simulink model "SecRwRtStLgrstInwdOtwdTrgtPosSelc"  (R2018b)
settings: Solver=FixedStepDiscrete  StartTime=0.0  StopTime=10.0  FixedStep=0.01  RelTol=1e-3
undefined symbols (not defined in the file or in its folder): KeSMSw4SAcsMd24SecRwRtStLegrstOtwdInwdPos_Val, KeSMSw4SAcsMd24SecRwRtStLegrstOtwdInwdPosMax_Val, KeSMSw4SAcsMd24SecRwRtStLegrstOtwdInwdPosMin_Val, KeSMSw4SAcsMd26SecRwRtStLegrstOtwdInwdPos_Val, KeSMSw4SAcsMd26SecRwRtStLegrstOtwdInwdPosMax_Val, KeSMSw4SAcsMd26SecRwRtStLegrstOtwdInwdPosMin_Val, KeSMSw4SLegrstCloseMdSecRwRtStLgrstOtwdInwdPos_Val, KeSMSw4SLegrstCloseMdSecRwRtStLgrstOtwdInwdPosMax_Val, KeSMSw4SLegrstCloseMdSecRwRtStLgrstOtwdInwdPosMin_Val, KeSMSw4SLegrstOpenMdSecRwRtStLgrstOtwdInwdPos_Val, KeSMSw4SLegrstOpenMdSecRwRtStLgrstOtwdInwdPosMax_Val, KeSMSw4SLegrstOpenMdSecRwRtStLgrstOtwdInwdPosMin_Val, KeSMSw4sLyingMDSecRwRtStLgrstOtwdInwdPos_160_Val, KeSMSw4sLyingMDSecRwRtStLgrstOtwdInwdPos_165_Val, KeSMSw4sLyingMDSecRwRtStLgrstOtwdInwdPos_170_Val, KeSMSw4sLyingMDSecRwRtStLgrstOtwdInwdPos_175_Val, KeSMSw4sLyingMDSecRwRtStLgrstOtwdInwdPos_180_Val, KeSMSw4sLyingMDSecRwRtStLgrstOtwdInwdPos_Below160_Val, KeSMSw4sLyingMDSecRwRtStLgrstOtwdInwdPos_Over180_Val, KeSMSw4sLyingMDSecRwRtStLgrstOtwdInwdPosMax_160_Val, KeSMSw4sLyingMDSecRwRtStLgrstOtwdInwdPosMax_165_Val, KeSMSw4sLyingMDSecRwRtStLgrstOtwdInwdPosMax_170_Val, KeSMSw4sLyingMDSecRwRtStLgrstOtwdInwdPosMax_175_Val, KeSMSw4sLyingMDSecRwRtStLgrstOtwdInwdPosMax_180_Val, KeSMSw4sLyingMDSecRwRtStLgrstOtwdInwdPosMax_Below160_Val, KeSMSw4sLyingMDSecRwRtStLgrstOtwdInwdPosMax_Over180_Val, KeSMSw4sLyingMDSecRwRtStLgrstOtwdInwdPosMin_160_Val, KeSMSw4sLyingMDSecRwRtStLgrstOtwdInwdPosMin_165_Val, KeSMSw4sLyingMDSecRwRtStLgrstOtwdInwdPosMin_170_Val, KeSMSw4sLyingMDSecRwRtStLgrstOtwdInwdPosMin_175_Val, KeSMSw4sLyingMDSecRwRtStLgrstOtwdInwdPosMin_180_Val, KeSMSw4sLyingMDSecRwRtStLgrstOtwdInwdPosMin_Below160_Val, KeSMSw4sLyingMDSecRwRtStLgrstOtwdInwdPosMin_Over180_Val, KeSMSw4sRecoveryMDSecRwRtStLgrstOtwdInwdPos_160_Val, KeSMSw4sRecoveryMDSecRwRtStLgrstOtwdInwdPos_165_Val, KeSMSw4sRecoveryMDSecRwRtStLgrstOtwdInwdPos_170_Val, KeSMSw4sRecoveryMDSecRwRtStLgrstOtwdInwdPos_175_Val, KeSMSw4sRecoveryMDSecRwRtStLgrstOtwdInwdPos_180_Val, KeSMSw4sRecoveryMDSecRwRtStLgrstOtwdInwdPos_Below160_Val, KeSMSw4sRecoveryMDSecRwRtStLgrstOtwdInwdPos_Over180_Val, KeSMSw4sRecoveryMDSecRwRtStLgrstOtwdInwdPosMax_160_Val, KeSMSw4sRecoveryMDSecRwRtStLgrstOtwdInwdPosMax_165_Val, KeSMSw4sRecoveryMDSecRwRtStLgrstOtwdInwdPosMax_170_Val, KeSMSw4sRecoveryMDSecRwRtStLgrstOtwdInwdPosMax_175_Val, KeSMSw4sRecoveryMDSecRwRtStLgrstOtwdInwdPosMax_180_Val, KeSMSw4sRecoveryMDSecRwRtStLgrstOtwdInwdPosMax_Below160_Val, KeSMSw4sRecoveryMDSecRwRtStLgrstOtwdInwdPosMax_Over180_Val, KeSMSw4sRecoveryMDSecRwRtStLgrstOtwdInwdPosMin_160_Val, KeSMSw4sRecoveryMDSecRwRtStLgrstOtwdInwdPosMin_165_Val, KeSMSw4sRecoveryMDSecRwRtStLgrstOtwdInwdPosMin_170_Val, KeSMSw4sRecoveryMDSecRwRtStLgrstOtwdInwdPosMin_175_Val, KeSMSw4sRecoveryMDSecRwRtStLgrstOtwdInwdPosMin_180_Val, KeSMSw4sRecoveryMDSecRwRtStLgrstOtwdInwdPosMin_Below160_Val, KeSMSw4sRecoveryMDSecRwRtStLgrstOtwdInwdPosMin_Over180_Val, KeSMSw4sVIPMDSecRwRtStLgrstOtwdInwdPos_160_Val, KeSMSw4sVIPMDSecRwRtStLgrstOtwdInwdPos_165_Val, KeSMSw4sVIPMDSecRwRtStLgrstOtwdInwdPos_170_Val, KeSMSw4sVIPMDSecRwRtStLgrstOtwdInwdPos_175_Val, KeSMSw4sVIPMDSecRwRtStLgrstOtwdInwdPos_180_Val, KeSMSw4sVIPMDSecRwRtStLgrstOtwdInwdPos_Below160_Val ... (+40)
libraries: TrgtPosSelcLib x10
(part 2 of 2)

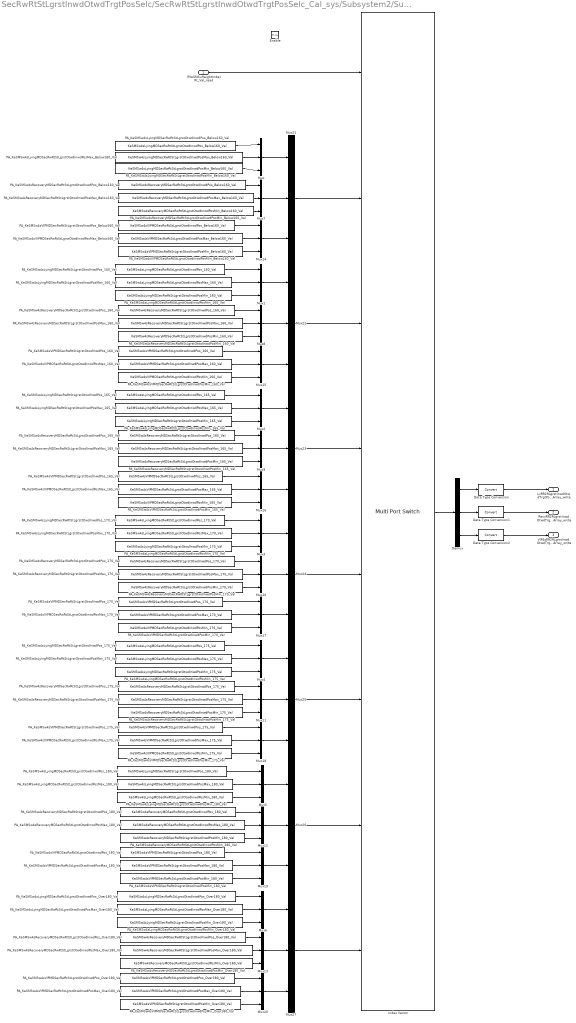
== system SecRwRtStLgrstInwdOtwdTrgtPosSelc/SecRwRtStLgrstInwdOtwdTrgtPosSelc_Cal_sys/Subsystem2/Subsystem ==
  IfVeSMSuHeightIndexRt_Val_read : Inport
  Enable : EnablePort
  Data Type Conversion : DataTypeConversion
  Data Type Conversion1 : DataTypeConversion
  Data Type Conversion2 : DataTypeConversion
  Demux : Demux  Outputs=3
  Index Vector : MultiPortSwitch  DataPortOrder=Zero-based contiguous  Inputs=7  zeroidx=on
  Mux{,1..27} (28 alike) : Mux  Inputs=3
  PA_KeSMSw4sLyingMDSecRwRtStLgrstOtwdInwdPosMax_160_Val : Constant  Value=KeSMSw4sLyingMDSecRwRtStLgrstOtwdInwdPosMax_160_Val
  PA_KeSMSw4sLyingMDSecRwRtStLgrstOtwdInwdPosMax_165_Val : Constant  Value=KeSMSw4sLyingMDSecRwRtStLgrstOtwdInwdPosMax_165_Val
  PA_KeSMSw4sLyingMDSecRwRtStLgrstOtwdInwdPosMax_170_Val : Constant  Value=KeSMSw4sLyingMDSecRwRtStLgrstOtwdInwdPosMax_170_Val
  PA_KeSMSw4sLyingMDSecRwRtStLgrstOtwdInwdPosMax_175_Val : Constant  Value=KeSMSw4sLyingMDSecRwRtStLgrstOtwdInwdPosMax_175_Val
  PA_KeSMSw4sLyingMDSecRwRtStLgrstOtwdInwdPosMax_180_Val : Constant  Value=KeSMSw4sLyingMDSecRwRtStLgrstOtwdInwdPosMax_180_Val
  PA_KeSMSw4sLyingMDSecRwRtStLgrstOtwdInwdPosMax_Below160_Val : Constant  Value=KeSMSw4sLyingMDSecRwRtStLgrstOtwdInwdPosMax_Below160_Val
  PA_KeSMSw4sLyingMDSecRwRtStLgrstOtwdInwdPosMax_Over180_Val : Constant  Value=KeSMSw4sLyingMDSecRwRtStLgrstOtwdInwdPosMax_Over180_Val
  PA_KeSMSw4sLyingMDSecRwRtStLgrstOtwdInwdPosMin_160_Val : Constant  Value=KeSMSw4sLyingMDSecRwRtStLgrstOtwdInwdPosMin_160_Val
  PA_KeSMSw4sLyingMDSecRwRtStLgrstOtwdInwdPosMin_165_Val : Constant  Value=KeSMSw4sLyingMDSecRwRtStLgrstOtwdInwdPosMin_165_Val
  PA_KeSMSw4sLyingMDSecRwRtStLgrstOtwdInwdPosMin_170_Val : Constant  Value=KeSMSw4sLyingMDSecRwRtStLgrstOtwdInwdPosMin_170_Val
  PA_KeSMSw4sLyingMDSecRwRtStLgrstOtwdInwdPosMin_175_Val : Constant  Value=KeSMSw4sLyingMDSecRwRtStLgrstOtwdInwdPosMin_175_Val
  PA_KeSMSw4sLyingMDSecRwRtStLgrstOtwdInwdPosMin_180_Val : Constant  Value=KeSMSw4sLyingMDSecRwRtStLgrstOtwdInwdPosMin_180_Val
  PA_KeSMSw4sLyingMDSecRwRtStLgrstOtwdInwdPosMin_Below160_Val : Constant  Value=KeSMSw4sLyingMDSecRwRtStLgrstOtwdInwdPosMin_Below160_Val
  PA_KeSMSw4sLyingMDSecRwRtStLgrstOtwdInwdPosMin_Over180_Val : Constant  Value=KeSMSw4sLyingMDSecRwRtStLgrstOtwdInwdPosMin_Over180_Val
  PA_KeSMSw4sLyingMDSecRwRtStLgrstOtwdInwdPos_160_Val : Constant  Value=KeSMSw4sLyingMDSecRwRtStLgrstOtwdInwdPos_160_Val
  PA_KeSMSw4sLyingMDSecRwRtStLgrstOtwdInwdPos_165_Val : Constant  Value=KeSMSw4sLyingMDSecRwRtStLgrstOtwdInwdPos_165_Val
  PA_KeSMSw4sLyingMDSecRwRtStLgrstOtwdInwdPos_170_Val : Constant  Value=KeSMSw4sLyingMDSecRwRtStLgrstOtwdInwdPos_170_Val
  PA_KeSMSw4sLyingMDSecRwRtStLgrstOtwdInwdPos_175_Val : Constant  Value=KeSMSw4sLyingMDSecRwRtStLgrstOtwdInwdPos_175_Val
  PA_KeSMSw4sLyingMDSecRwRtStLgrstOtwdInwdPos_180_Val : Constant  Value=KeSMSw4sLyingMDSecRwRtStLgrstOtwdInwdPos_180_Val
  PA_KeSMSw4sLyingMDSecRwRtStLgrstOtwdInwdPos_Below160_Val : Constant  Value=KeSMSw4sLyingMDSecRwRtStLgrstOtwdInwdPos_Below160_Val
  PA_KeSMSw4sLyingMDSecRwRtStLgrstOtwdInwdPos_Over180_Val : Constant  Value=KeSMSw4sLyingMDSecRwRtStLgrstOtwdInwdPos_Over180_Val
  PA_KeSMSw4sRecoveryMDSecRwRtStLgrstOtwdInwdPosMax_160_Val : Constant  Value=KeSMSw4sRecoveryMDSecRwRtStLgrstOtwdInwdPosMax_160_Val
  PA_KeSMSw4sRecoveryMDSecRwRtStLgrstOtwdInwdPosMax_165_Val : Constant  Value=KeSMSw4sRecoveryMDSecRwRtStLgrstOtwdInwdPosMax_165_Val
  PA_KeSMSw4sRecoveryMDSecRwRtStLgrstOtwdInwdPosMax_170_Val : Constant  Value=KeSMSw4sRecoveryMDSecRwRtStLgrstOtwdInwdPosMax_170_Val
  PA_KeSMSw4sRecoveryMDSecRwRtStLgrstOtwdInwdPosMax_175_Val : Constant  Value=KeSMSw4sRecoveryMDSecRwRtStLgrstOtwdInwdPosMax_175_Val
  PA_KeSMSw4sRecoveryMDSecRwRtStLgrstOtwdInwdPosMax_180_Val : Constant  Value=KeSMSw4sRecoveryMDSecRwRtStLgrstOtwdInwdPosMax_180_Val
  PA_KeSMSw4sRecoveryMDSecRwRtStLgrstOtwdInwdPosMax_Below160_Val : Constant  Value=KeSMSw4sRecoveryMDSecRwRtStLgrstOtwdInwdPosMax_Below160_Val
  PA_KeSMSw4sRecoveryMDSecRwRtStLgrstOtwdInwdPosMax_Over180_Val : Constant  Value=KeSMSw4sRecoveryMDSecRwRtStLgrstOtwdInwdPosMax_Over180_Val
  PA_KeSMSw4sRecoveryMDSecRwRtStLgrstOtwdInwdPosMin_160_Val : Constant  Value=KeSMSw4sRecoveryMDSecRwRtStLgrstOtwdInwdPosMin_160_Val
  PA_KeSMSw4sRecoveryMDSecRwRtStLgrstOtwdInwdPosMin_165_Val : Constant  Value=KeSMSw4sRecoveryMDSecRwRtStLgrstOtwdInwdPosMin_165_Val
  PA_KeSMSw4sRecoveryMDSecRwRtStLgrstOtwdInwdPosMin_170_Val : Constant  Value=KeSMSw4sRecoveryMDSecRwRtStLgrstOtwdInwdPosMin_170_Val
  PA_KeSMSw4sRecoveryMDSecRwRtStLgrstOtwdInwdPosMin_175_Val : Constant  Value=KeSMSw4sRecoveryMDSecRwRtStLgrstOtwdInwdPosMin_175_Val
  PA_KeSMSw4sRecoveryMDSecRwRtStLgrstOtwdInwdPosMin_180_Val : Constant  Value=KeSMSw4sRecoveryMDSecRwRtStLgrstOtwdInwdPosMin_180_Val
  PA_KeSMSw4sRecoveryMDSecRwRtStLgrstOtwdInwdPosMin_Below160_Val : Constant  Value=KeSMSw4sRecoveryMDSecRwRtStLgrstOtwdInwdPosMin_Below160_Val
  PA_KeSMSw4sRecoveryMDSecRwRtStLgrstOtwdInwdPosMin_Over180_Val : Constant  Value=KeSMSw4sRecoveryMDSecRwRtStLgrstOtwdInwdPosMin_Over180_Val
  PA_KeSMSw4sRecoveryMDSecRwRtStLgrstOtwdInwdPos_160_Val : Constant  Value=KeSMSw4sRecoveryMDSecRwRtStLgrstOtwdInwdPos_160_Val
  PA_KeSMSw4sRecoveryMDSecRwRtStLgrstOtwdInwdPos_165_Val : Constant  Value=KeSMSw4sRecoveryMDSecRwRtStLgrstOtwdInwdPos_165_Val
  PA_KeSMSw4sRecoveryMDSecRwRtStLgrstOtwdInwdPos_170_Val : Constant  Value=KeSMSw4sRecoveryMDSecRwRtStLgrstOtwdInwdPos_170_Val
  PA_KeSMSw4sRecoveryMDSecRwRtStLgrstOtwdInwdPos_175_Val : Constant  Value=KeSMSw4sRecoveryMDSecRwRtStLgrstOtwdInwdPos_175_Val
  PA_KeSMSw4sRecoveryMDSecRwRtStLgrstOtwdInwdPos_180_Val : Constant  Value=KeSMSw4sRecoveryMDSecRwRtStLgrstOtwdInwdPos_180_Val
  PA_KeSMSw4sRecoveryMDSecRwRtStLgrstOtwdInwdPos_Below160_Val : Constant  Value=KeSMSw4sRecoveryMDSecRwRtStLgrstOtwdInwdPos_Below160_Val
  PA_KeSMSw4sRecoveryMDSecRwRtStLgrstOtwdInwdPos_Over180_Val : Constant  Value=KeSMSw4sRecoveryMDSecRwRtStLgrstOtwdInwdPos_Over180_Val
  PA_KeSMSw4sVIPMDSecRwRtStLgrstOtwdInwdPosMax_160_Val : Constant  Value=KeSMSw4sVIPMDSecRwRtStLgrstOtwdInwdPosMax_160_Val
  PA_KeSMSw4sVIPMDSecRwRtStLgrstOtwdInwdPosMax_165_Val : Constant  Value=KeSMSw4sVIPMDSecRwRtStLgrstOtwdInwdPosMax_165_Val
  PA_KeSMSw4sVIPMDSecRwRtStLgrstOtwdInwdPosMax_170_Val : Constant  Value=KeSMSw4sVIPMDSecRwRtStLgrstOtwdInwdPosMax_170_Val
  PA_KeSMSw4sVIPMDSecRwRtStLgrstOtwdInwdPosMax_175_Val : Constant  Value=KeSMSw4sVIPMDSecRwRtStLgrstOtwdInwdPosMax_175_Val
  PA_KeSMSw4sVIPMDSecRwRtStLgrstOtwdInwdPosMax_180_Val : Constant  Value=KeSMSw4sVIPMDSecRwRtStLgrstOtwdInwdPosMax_180_Val
  PA_KeSMSw4sVIPMDSecRwRtStLgrstOtwdInwdPosMax_Below160_Val : Constant  Value=KeSMSw4sVIPMDSecRwRtStLgrstOtwdInwdPosMax_Below160_Val
  PA_KeSMSw4sVIPMDSecRwRtStLgrstOtwdInwdPosMax_Over180_Val : Constant  Value=KeSMSw4sVIPMDSecRwRtStLgrstOtwdInwdPosMax_Over180_Val
  PA_KeSMSw4sVIPMDSecRwRtStLgrstOtwdInwdPosMin_160_Val : Constant  Value=KeSMSw4sVIPMDSecRwRtStLgrstOtwdInwdPosMin_160_Val
  PA_KeSMSw4sVIPMDSecRwRtStLgrstOtwdInwdPosMin_165_Val : Constant  Value=KeSMSw4sVIPMDSecRwRtStLgrstOtwdInwdPosMin_165_Val
  PA_KeSMSw4sVIPMDSecRwRtStLgrstOtwdInwdPosMin_170_Val : Constant  Value=KeSMSw4sVIPMDSecRwRtStLgrstOtwdInwdPosMin_170_Val
  PA_KeSMSw4sVIPMDSecRwRtStLgrstOtwdInwdPosMin_175_Val : Constant  Value=KeSMSw4sVIPMDSecRwRtStLgrstOtwdInwdPosMin_175_Val
  PA_KeSMSw4sVIPMDSecRwRtStLgrstOtwdInwdPosMin_180_Val : Constant  Value=KeSMSw4sVIPMDSecRwRtStLgrstOtwdInwdPosMin_180_Val
  PA_KeSMSw4sVIPMDSecRwRtStLgrstOtwdInwdPosMin_Below160_Val : Constant  Value=KeSMSw4sVIPMDSecRwRtStLgrstOtwdInwdPosMin_Below160_Val
  PA_KeSMSw4sVIPMDSecRwRtStLgrstOtwdInwdPosMin_Over180_Val : Constant  Value=KeSMSw4sVIPMDSecRwRtStLgrstOtwdInwdPosMin_Over180_Val
  PA_KeSMSw4sVIPMDSecRwRtStLgrstOtwdInwdPos_160_Val : Constant  Value=KeSMSw4sVIPMDSecRwRtStLgrstOtwdInwdPos_160_Val
  PA_KeSMSw4sVIPMDSecRwRtStLgrstOtwdInwdPos_165_Val : Constant  Value=KeSMSw4sVIPMDSecRwRtStLgrstOtwdInwdPos_165_Val
  PA_KeSMSw4sVIPMDSecRwRtStLgrstOtwdInwdPos_170_Val : Constant  Value=KeSMSw4sVIPMDSecRwRtStLgrstOtwdInwdPos_170_Val
  PA_KeSMSw4sVIPMDSecRwRtStLgrstOtwdInwdPos_175_Val : Constant  Value=KeSMSw4sVIPMDSecRwRtStLgrstOtwdInwdPos_175_Val
  PA_KeSMSw4sVIPMDSecRwRtStLgrstOtwdInwdPos_180_Val : Constant  Value=KeSMSw4sVIPMDSecRwRtStLgrstOtwdInwdPos_180_Val
  PA_KeSMSw4sVIPMDSecRwRtStLgrstOtwdInwdPos_Below160_Val : Constant  Value=KeSMSw4sVIPMDSecRwRtStLgrstOtwdInwdPos_Below160_Val
  PA_KeSMSw4sVIPMDSecRwRtStLgrstOtwdInwdPos_Over180_Val : Constant  Value=KeSMSw4sVIPMDSecRwRtStLgrstOtwdInwdPos_Over180_Val
  LyRR2RLgrstInwdOtwdTrgtPosCalib_TrgtPosArray_write : Outport
  RecvRR2RLgrstInwdOtwdTrgtPosCalib_TrgtPosArray_write : Outport  Port=2
  VIP4sRR2RLgrstInwdOtwdTrgtPosCalib_TrgtPosArray_write : Outport  Port=3
  wires:
  Demux/1 -> Data Type Conversion/1
  Demux/2 -> Data Type Conversion1/1
  Demux/3 -> Data Type Conversion2/1
  Data Type Conversion/1 -> LyRR2RLgrstInwdOtwdTrgtPosCalib_TrgtPosArray_write/1
  Data Type Conversion1/1 -> RecvRR2RLgrstInwdOtwdTrgtPosCalib_TrgtPosArray_write/1
  Data Type Conversion2/1 -> VIP4sRR2RLgrstInwdOtwdTrgtPosCalib_TrgtPosArray_write/1
  PA_KeSMSw4sLyingMDSecRwRtStLgrstOtwdInwdPosMax_Below160_Val/1 -> Mux/2
  PA_KeSMSw4sLyingMDSecRwRtStLgrstOtwdInwdPosMin_Below160_Val/1 -> Mux/3
  PA_KeSMSw4sLyingMDSecRwRtStLgrstOtwdInwdPos_Below160_Val/1 -> Mux/1
  PA_KeSMSw4sLyingMDSecRwRtStLgrstOtwdInwdPosMax_160_Val/1 -> Mux1/2
  PA_KeSMSw4sLyingMDSecRwRtStLgrstOtwdInwdPosMin_160_Val/1 -> Mux1/3
  PA_KeSMSw4sLyingMDSecRwRtStLgrstOtwdInwdPos_160_Val/1 -> Mux1/1
  PA_KeSMSw4sLyingMDSecRwRtStLgrstOtwdInwdPosMax_165_Val/1 -> Mux2/2
  PA_KeSMSw4sLyingMDSecRwRtStLgrstOtwdInwdPosMin_165_Val/1 -> Mux2/3
  PA_KeSMSw4sLyingMDSecRwRtStLgrstOtwdInwdPos_165_Val/1 -> Mux2/1
  PA_KeSMSw4sLyingMDSecRwRtStLgrstOtwdInwdPosMax_170_Val/1 -> Mux3/2
  PA_KeSMSw4sLyingMDSecRwRtStLgrstOtwdInwdPosMin_170_Val/1 -> Mux3/3
  PA_KeSMSw4sLyingMDSecRwRtStLgrstOtwdInwdPos_170_Val/1 -> Mux3/1
  PA_KeSMSw4sLyingMDSecRwRtStLgrstOtwdInwdPosMax_175_Val/1 -> Mux4/2
  PA_KeSMSw4sLyingMDSecRwRtStLgrstOtwdInwdPosMin_175_Val/1 -> Mux4/3
  PA_KeSMSw4sLyingMDSecRwRtStLgrstOtwdInwdPos_175_Val/1 -> Mux4/1
  PA_KeSMSw4sLyingMDSecRwRtStLgrstOtwdInwdPosMax_180_Val/1 -> Mux5/2
  PA_KeSMSw4sLyingMDSecRwRtStLgrstOtwdInwdPosMin_180_Val/1 -> Mux5/3
  PA_KeSMSw4sLyingMDSecRwRtStLgrstOtwdInwdPos_180_Val/1 -> Mux5/1
  PA_KeSMSw4sLyingMDSecRwRtStLgrstOtwdInwdPosMax_Over180_Val/1 -> Mux6/2
  PA_KeSMSw4sLyingMDSecRwRtStLgrstOtwdInwdPosMin_Over180_Val/1 -> Mux6/3
  PA_KeSMSw4sLyingMDSecRwRtStLgrstOtwdInwdPos_Over180_Val/1 -> Mux6/1
  IfVeSMSuHeightIndexRt_Val_read/1 -> Index Vector/1
  PA_KeSMSw4sRecoveryMDSecRwRtStLgrstOtwdInwdPos_Below160_Val/1 -> Mux7/1
  PA_KeSMSw4sRecoveryMDSecRwRtStLgrstOtwdInwdPosMax_Below160_Val/1 -> Mux7/2
  PA_KeSMSw4sRecoveryMDSecRwRtStLgrstOtwdInwdPosMin_Below160_Val/1 -> Mux7/3
  PA_KeSMSw4sRecoveryMDSecRwRtStLgrstOtwdInwdPos_160_Val/1 -> Mux8/1
  PA_KeSMSw4sRecoveryMDSecRwRtStLgrstOtwdInwdPosMax_160_Val/1 -> Mux8/2
  PA_KeSMSw4sRecoveryMDSecRwRtStLgrstOtwdInwdPosMin_160_Val/1 -> Mux8/3
  PA_KeSMSw4sRecoveryMDSecRwRtStLgrstOtwdInwdPos_165_Val/1 -> Mux9/1
  PA_KeSMSw4sRecoveryMDSecRwRtStLgrstOtwdInwdPosMax_165_Val/1 -> Mux9/2
  PA_KeSMSw4sRecoveryMDSecRwRtStLgrstOtwdInwdPosMin_165_Val/1 -> Mux9/3
  PA_KeSMSw4sRecoveryMDSecRwRtStLgrstOtwdInwdPos_170_Val/1 -> Mux10/1
  PA_KeSMSw4sRecoveryMDSecRwRtStLgrstOtwdInwdPosMax_170_Val/1 -> Mux10/2
  PA_KeSMSw4sRecoveryMDSecRwRtStLgrstOtwdInwdPosMin_170_Val/1 -> Mux10/3
  PA_KeSMSw4sRecoveryMDSecRwRtStLgrstOtwdInwdPos_175_Val/1 -> Mux11/1
  PA_KeSMSw4sRecoveryMDSecRwRtStLgrstOtwdInwdPosMax_175_Val/1 -> Mux11/2
  PA_KeSMSw4sRecoveryMDSecRwRtStLgrstOtwdInwdPosMin_175_Val/1 -> Mux11/3
  PA_KeSMSw4sRecoveryMDSecRwRtStLgrstOtwdInwdPos_180_Val/1 -> Mux12/1
  PA_KeSMSw4sRecoveryMDSecRwRtStLgrstOtwdInwdPosMax_180_Val/1 -> Mux12/2
  PA_KeSMSw4sRecoveryMDSecRwRtStLgrstOtwdInwdPosMin_180_Val/1 -> Mux12/3
  PA_KeSMSw4sRecoveryMDSecRwRtStLgrstOtwdInwdPos_Over180_Val/1 -> Mux13/1
  PA_KeSMSw4sRecoveryMDSecRwRtStLgrstOtwdInwdPosMax_Over180_Val/1 -> Mux13/2
  PA_KeSMSw4sRecoveryMDSecRwRtStLgrstOtwdInwdPosMin_Over180_Val/1 -> Mux13/3
  PA_KeSMSw4sVIPMDSecRwRtStLgrstOtwdInwdPos_Below160_Val/1 -> Mux14/1
  PA_KeSMSw4sVIPMDSecRwRtStLgrstOtwdInwdPosMax_Below160_Val/1 -> Mux14/2
  PA_KeSMSw4sVIPMDSecRwRtStLgrstOtwdInwdPosMin_Below160_Val/1 -> Mux14/3
  PA_KeSMSw4sVIPMDSecRwRtStLgrstOtwdInwdPos_160_Val/1 -> Mux15/1
  PA_KeSMSw4sVIPMDSecRwRtStLgrstOtwdInwdPosMax_160_Val/1 -> Mux15/2
  PA_KeSMSw4sVIPMDSecRwRtStLgrstOtwdInwdPosMin_160_Val/1 -> Mux15/3
  PA_KeSMSw4sVIPMDSecRwRtStLgrstOtwdInwdPos_165_Val/1 -> Mux16/1
  PA_KeSMSw4sVIPMDSecRwRtStLgrstOtwdInwdPosMax_165_Val/1 -> Mux16/2
  PA_KeSMSw4sVIPMDSecRwRtStLgrstOtwdInwdPosMin_165_Val/1 -> Mux16/3
  PA_KeSMSw4sVIPMDSecRwRtStLgrstOtwdInwdPos_170_Val/1 -> Mux17/1
  PA_KeSMSw4sVIPMDSecRwRtStLgrstOtwdInwdPosMax_170_Val/1 -> Mux17/2
  PA_KeSMSw4sVIPMDSecRwRtStLgrstOtwdInwdPosMin_170_Val/1 -> Mux17/3
  PA_KeSMSw4sVIPMDSecRwRtStLgrstOtwdInwdPos_175_Val/1 -> Mux18/1
  PA_KeSMSw4sVIPMDSecRwRtStLgrstOtwdInwdPosMax_175_Val/1 -> Mux18/2
  PA_KeSMSw4sVIPMDSecRwRtStLgrstOtwdInwdPosMin_175_Val/1 -> Mux18/3
  PA_KeSMSw4sVIPMDSecRwRtStLgrstOtwdInwdPos_180_Val/1 -> Mux19/1
  PA_KeSMSw4sVIPMDSecRwRtStLgrstOtwdInwdPosMax_180_Val/1 -> Mux19/2
  PA_KeSMSw4sVIPMDSecRwRtStLgrstOtwdInwdPosMin_180_Val/1 -> Mux19/3
  PA_KeSMSw4sVIPMDSecRwRtStLgrstOtwdInwdPos_Over180_Val/1 -> Mux20/1
  PA_KeSMSw4sVIPMDSecRwRtStLgrstOtwdInwdPosMax_Over180_Val/1 -> Mux20/2
  PA_KeSMSw4sVIPMDSecRwRtStLgrstOtwdInwdPosMin_Over180_Val/1 -> Mux20/3
  Mux21/1 -> Index Vector/2
  Mux22/1 -> Index Vector/3
  Mux/1 -> Mux21/1
  Mux7/1 -> Mux21/2
  Mux14/1 -> Mux21/3
  Mux23/1 -> Index Vector/4
  Mux24/1 -> Index Vector/5
  Mux25/1 -> Index Vector/6
  Mux26/1 -> Index Vector/7
  Mux27/1 -> Index Vector/8
  Mux1/1 -> Mux22/1
  Mux8/1 -> Mux22/2
  Mux15/1 -> Mux22/3
  Mux2/1 -> Mux23/1
  Mux9/1 -> Mux23/2
  Mux16/1 -> Mux23/3
  Mux3/1 -> Mux24/1
  Mux10/1 -> Mux24/2
  Mux17/1 -> Mux24/3
  Mux4/1 -> Mux25/1
  Mux11/1 -> Mux25/2
  Mux18/1 -> Mux25/3
  Mux5/1 -> Mux26/1
  Mux12/1 -> Mux26/2
  Mux19/1 -> Mux26/3
  Mux6/1 -> Mux27/1
  Mux13/1 -> Mux27/2
  Mux20/1 -> Mux27/3
  Index Vector/1 -> Demux/1

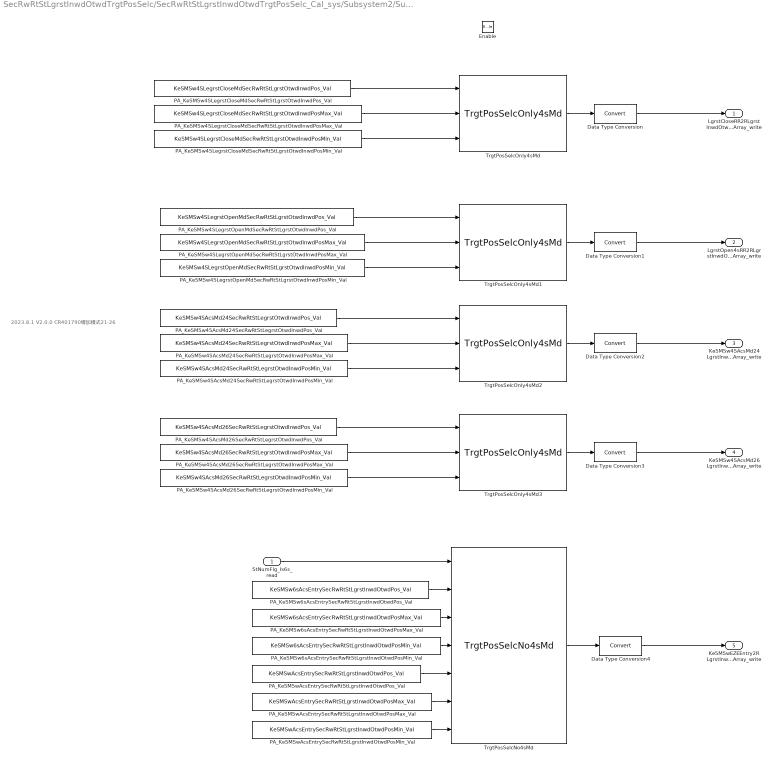
== system SecRwRtStLgrstInwdOtwdTrgtPosSelc/SecRwRtStLgrstInwdOtwdTrgtPosSelc_Cal_sys/Subsystem2/Subsystem1 ==
  note: 2023.8.1 V2.0.0 CR401790 增加模式21-26
  StNumFlg_Is6s_read : Inport
  Enable : EnablePort
  Data Type Conversion{,1..4} (5 alike) : DataTypeConversion
  PA_KeSMSw4SAcsMd24SecRwRtStLegrstOtwdInwdPosMax_Val : Constant  Value=KeSMSw4SAcsMd24SecRwRtStLegrstOtwdInwdPosMax_Val
  PA_KeSMSw4SAcsMd24SecRwRtStLegrstOtwdInwdPosMin_Val : Constant  Value=KeSMSw4SAcsMd24SecRwRtStLegrstOtwdInwdPosMin_Val
  PA_KeSMSw4SAcsMd24SecRwRtStLegrstOtwdInwdPos_Val : Constant  Value=KeSMSw4SAcsMd24SecRwRtStLegrstOtwdInwdPos_Val
  PA_KeSMSw4SAcsMd26SecRwRtStLegrstOtwdInwdPosMax_Val : Constant  Value=KeSMSw4SAcsMd26SecRwRtStLegrstOtwdInwdPosMax_Val
  PA_KeSMSw4SAcsMd26SecRwRtStLegrstOtwdInwdPosMin_Val : Constant  Value=KeSMSw4SAcsMd26SecRwRtStLegrstOtwdInwdPosMin_Val
  PA_KeSMSw4SAcsMd26SecRwRtStLegrstOtwdInwdPos_Val : Constant  Value=KeSMSw4SAcsMd26SecRwRtStLegrstOtwdInwdPos_Val
  PA_KeSMSw4SLegrstCloseMdSecRwRtStLgrstOtwdInwdPosMax_Val : Constant  Value=KeSMSw4SLegrstCloseMdSecRwRtStLgrstOtwdInwdPosMax_Val
  PA_KeSMSw4SLegrstCloseMdSecRwRtStLgrstOtwdInwdPosMin_Val : Constant  Value=KeSMSw4SLegrstCloseMdSecRwRtStLgrstOtwdInwdPosMin_Val
  PA_KeSMSw4SLegrstCloseMdSecRwRtStLgrstOtwdInwdPos_Val : Constant  Value=KeSMSw4SLegrstCloseMdSecRwRtStLgrstOtwdInwdPos_Val
  PA_KeSMSw4SLegrstOpenMdSecRwRtStLgrstOtwdInwdPosMax_Val : Constant  Value=KeSMSw4SLegrstOpenMdSecRwRtStLgrstOtwdInwdPosMax_Val
  PA_KeSMSw4SLegrstOpenMdSecRwRtStLgrstOtwdInwdPosMin_Val : Constant  Value=KeSMSw4SLegrstOpenMdSecRwRtStLgrstOtwdInwdPosMin_Val
  PA_KeSMSw4SLegrstOpenMdSecRwRtStLgrstOtwdInwdPos_Val : Constant  Value=KeSMSw4SLegrstOpenMdSecRwRtStLgrstOtwdInwdPos_Val
  PA_KeSMSw6sAcsEntrySecRwRtStLgrstInwdOtwdPosMax_Val : Constant  Value=KeSMSw6sAcsEntrySecRwRtStLgrstInwdOtwdPosMax_Val
  PA_KeSMSw6sAcsEntrySecRwRtStLgrstInwdOtwdPosMin_Val : Constant  Value=KeSMSw6sAcsEntrySecRwRtStLgrstInwdOtwdPosMin_Val
  PA_KeSMSw6sAcsEntrySecRwRtStLgrstInwdOtwdPos_Val : Constant  Value=KeSMSw6sAcsEntrySecRwRtStLgrstInwdOtwdPos_Val
  PA_KeSMSwAcsEntrySecRwRtStLgrstInwdOtwdPosMax_Val : Constant  Value=KeSMSwAcsEntrySecRwRtStLgrstInwdOtwdPosMax_Val
  PA_KeSMSwAcsEntrySecRwRtStLgrstInwdOtwdPosMin_Val : Constant  Value=KeSMSwAcsEntrySecRwRtStLgrstInwdOtwdPosMin_Val
  PA_KeSMSwAcsEntrySecRwRtStLgrstInwdOtwdPos_Val : Constant  Value=KeSMSwAcsEntrySecRwRtStLgrstInwdOtwdPos_Val
  TrgtPosSelcNo4sMd : TrgtPosSelcLib/TrgtPosSelcNo4sMd  SystemSampleTime=-1
  TrgtPosSelcOnly4sMd{,1..3} (4 alike) : TrgtPosSelcLib/TrgtPosSelcOnly4sMd  SystemSampleTime=-1
  LgrstCloseRR2RLgrstInwdOtwdTrgtPosCalib_TrgtPosArray_write : Outport
  LgrstOpen4sRR2RLgrstInwdOtwdTrgtPosCalib_TrgtPosArray_write : Outport  Port=2
  KeSMSw4SAcsMd24LgrstInwdOtwdTrgtPosCalib_TrgtPosArray_write : Outport  Port=3
  KeSMSw4SAcsMd26LgrstInwdOtwdTrgtPosCalib_TrgtPosArray_write : Outport  Port=4
  KeSMSwEZEEntry2RLgrstInwdOtwdTrgtPosCalib_TrgtPosArray_write : Outport  Port=5
  wires:
  TrgtPosSelcOnly4sMd1/1 -> Data Type Conversion1/1
  PA_KeSMSw4SLegrstOpenMdSecRwRtStLgrstOtwdInwdPosMin_Val/1 -> TrgtPosSelcOnly4sMd1/3
  PA_KeSMSw4SLegrstOpenMdSecRwRtStLgrstOtwdInwdPosMax_Val/1 -> TrgtPosSelcOnly4sMd1/2
  TrgtPosSelcOnly4sMd/1 -> Data Type Conversion/1
  PA_KeSMSw4SLegrstOpenMdSecRwRtStLgrstOtwdInwdPos_Val/1 -> TrgtPosSelcOnly4sMd1/1
  PA_KeSMSw4SLegrstCloseMdSecRwRtStLgrstOtwdInwdPos_Val/1 -> TrgtPosSelcOnly4sMd/1
  PA_KeSMSw4SLegrstCloseMdSecRwRtStLgrstOtwdInwdPosMax_Val/1 -> TrgtPosSelcOnly4sMd/2
  PA_KeSMSw4SLegrstCloseMdSecRwRtStLgrstOtwdInwdPosMin_Val/1 -> TrgtPosSelcOnly4sMd/3
  Data Type Conversion/1 -> LgrstCloseRR2RLgrstInwdOtwdTrgtPosCalib_TrgtPosArray_write/1
  Data Type Conversion1/1 -> LgrstOpen4sRR2RLgrstInwdOtwdTrgtPosCalib_TrgtPosArray_write/1
  TrgtPosSelcOnly4sMd2/1 -> Data Type Conversion2/1
  TrgtPosSelcOnly4sMd3/1 -> Data Type Conversion3/1
  Data Type Conversion2/1 -> KeSMSw4SAcsMd24LgrstInwdOtwdTrgtPosCalib_TrgtPosArray_write/1
  Data Type Conversion3/1 -> KeSMSw4SAcsMd26LgrstInwdOtwdTrgtPosCalib_TrgtPosArray_write/1
  PA_KeSMSw4SAcsMd24SecRwRtStLegrstOtwdInwdPosMax_Val/1 -> TrgtPosSelcOnly4sMd2/2
  PA_KeSMSw4SAcsMd24SecRwRtStLegrstOtwdInwdPosMin_Val/1 -> TrgtPosSelcOnly4sMd2/3
  PA_KeSMSw4SAcsMd24SecRwRtStLegrstOtwdInwdPos_Val/1 -> TrgtPosSelcOnly4sMd2/1
  PA_KeSMSw4SAcsMd26SecRwRtStLegrstOtwdInwdPosMax_Val/1 -> TrgtPosSelcOnly4sMd3/2
  PA_KeSMSw4SAcsMd26SecRwRtStLegrstOtwdInwdPosMin_Val/1 -> TrgtPosSelcOnly4sMd3/3
  PA_KeSMSw4SAcsMd26SecRwRtStLegrstOtwdInwdPos_Val/1 -> TrgtPosSelcOnly4sMd3/1
  TrgtPosSelcNo4sMd/1 -> Data Type Conversion4/1
  Data Type Conversion4/1 -> KeSMSwEZEEntry2RLgrstInwdOtwdTrgtPosCalib_TrgtPosArray_write/1
  StNumFlg_Is6s_read/1 -> TrgtPosSelcNo4sMd/1
  PA_KeSMSw6sAcsEntrySecRwRtStLgrstInwdOtwdPos_Val/1 -> TrgtPosSelcNo4sMd/2
  PA_KeSMSw6sAcsEntrySecRwRtStLgrstInwdOtwdPosMax_Val/1 -> TrgtPosSelcNo4sMd/3
  PA_KeSMSw6sAcsEntrySecRwRtStLgrstInwdOtwdPosMin_Val/1 -> TrgtPosSelcNo4sMd/4
  PA_KeSMSwAcsEntrySecRwRtStLgrstInwdOtwdPos_Val/1 -> TrgtPosSelcNo4sMd/5
  PA_KeSMSwAcsEntrySecRwRtStLgrstInwdOtwdPosMax_Val/1 -> TrgtPosSelcNo4sMd/6
  PA_KeSMSwAcsEntrySecRwRtStLgrstInwdOtwdPosMin_Val/1 -> TrgtPosSelcNo4sMd/7

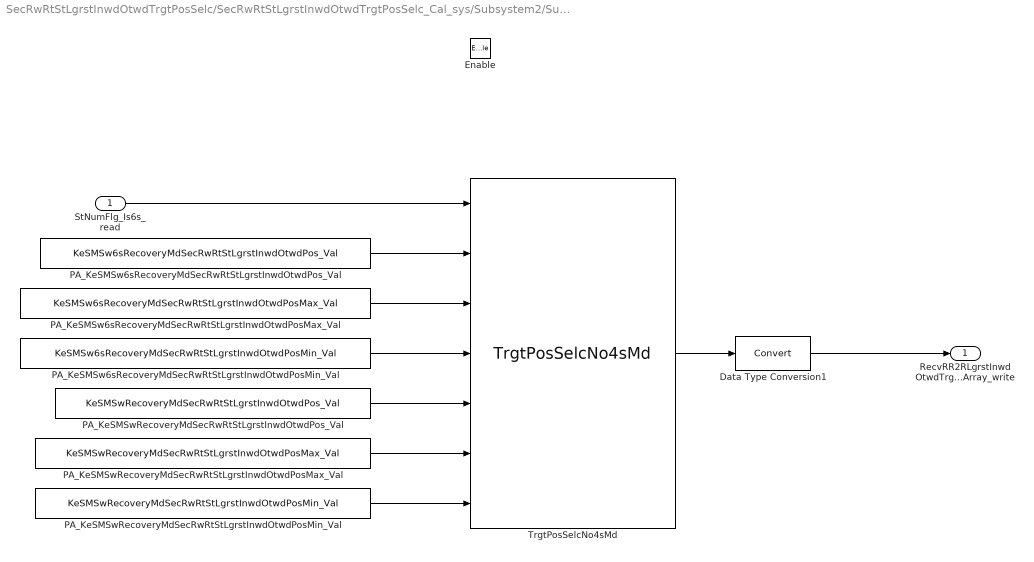
== system SecRwRtStLgrstInwdOtwdTrgtPosSelc/SecRwRtStLgrstInwdOtwdTrgtPosSelc_Cal_sys/Subsystem2/Subsystem2 ==
  StNumFlg_Is6s_read : Inport
  Enable : EnablePort
  Data Type Conversion1 : DataTypeConversion
  PA_KeSMSw6sRecoveryMdSecRwRtStLgrstInwdOtwdPosMax_Val : Constant  Value=KeSMSw6sRecoveryMdSecRwRtStLgrstInwdOtwdPosMax_Val
  PA_KeSMSw6sRecoveryMdSecRwRtStLgrstInwdOtwdPosMin_Val : Constant  Value=KeSMSw6sRecoveryMdSecRwRtStLgrstInwdOtwdPosMin_Val
  PA_KeSMSw6sRecoveryMdSecRwRtStLgrstInwdOtwdPos_Val : Constant  Value=KeSMSw6sRecoveryMdSecRwRtStLgrstInwdOtwdPos_Val
  PA_KeSMSwRecoveryMdSecRwRtStLgrstInwdOtwdPosMax_Val : Constant  Value=KeSMSwRecoveryMdSecRwRtStLgrstInwdOtwdPosMax_Val
  PA_KeSMSwRecoveryMdSecRwRtStLgrstInwdOtwdPosMin_Val : Constant  Value=KeSMSwRecoveryMdSecRwRtStLgrstInwdOtwdPosMin_Val
  PA_KeSMSwRecoveryMdSecRwRtStLgrstInwdOtwdPos_Val : Constant  Value=KeSMSwRecoveryMdSecRwRtStLgrstInwdOtwdPos_Val
  TrgtPosSelcNo4sMd : TrgtPosSelcLib/TrgtPosSelcNo4sMd  SystemSampleTime=-1
  RecvRR2RLgrstInwdOtwdTrgtPosCalib_TrgtPosArray_write : Outport
  wires:
  TrgtPosSelcNo4sMd/1 -> Data Type Conversion1/1
  StNumFlg_Is6s_read/1 -> TrgtPosSelcNo4sMd/1
  PA_KeSMSw6sRecoveryMdSecRwRtStLgrstInwdOtwdPos_Val/1 -> TrgtPosSelcNo4sMd/2
  PA_KeSMSw6sRecoveryMdSecRwRtStLgrstInwdOtwdPosMax_Val/1 -> TrgtPosSelcNo4sMd/3
  PA_KeSMSw6sRecoveryMdSecRwRtStLgrstInwdOtwdPosMin_Val/1 -> TrgtPosSelcNo4sMd/4
  PA_KeSMSwRecoveryMdSecRwRtStLgrstInwdOtwdPos_Val/1 -> TrgtPosSelcNo4sMd/5
  PA_KeSMSwRecoveryMdSecRwRtStLgrstInwdOtwdPosMax_Val/1 -> TrgtPosSelcNo4sMd/6
  PA_KeSMSwRecoveryMdSecRwRtStLgrstInwdOtwdPosMin_Val/1 -> TrgtPosSelcNo4sMd/7
  Data Type Conversion1/1 -> RecvRR2RLgrstInwdOtwdTrgtPosCalib_TrgtPosArray_write/1
